simulink model "transmission"  (R2020a)
settings: Solver=ode45  StartTime=0.0  StopTime=30.0  MaxStep=0.05  RelTol=1e-3  EnableMultiTasking=on
model workspace (MAT data in the model file):
  Cd = 0.02
  F = 40
  Ie = 0.0219914882836
  Iv = 12.0941478573
  K = [137.465208994; 137.065019157; 135.864449646; 135.664354728; 137.565256453; 140.366585312; 145.268910814; 152.872517717; 162.9773111; 164.27792807; 166.178829795; 167.979684062; 170.080680706; 172.781962105; 175.383196045; 179.585189333; 183.587087703; 189.890077635; 197.693779455; 215.902417037; 244.515990379]
  Ne = [800 1200 1600 2000 2400 2800 3200 3600 4000 4400 4800]
  Qfd = 3.23
  Qn = [0; 0.1; 0.2; 0.3; 0.4; 0.5; 0.6; 0.7; 0.8; 0.81; 0.82; 0.83; 0.84; 0.85; 0.86; 0.87; 0.88; 0.89; 0.9; 0.92; 0.94]
  Qt = [2.232; 2.075; 1.975; 1.846; 1.72; 1.564; 1.409; 1.254; 1.096; 1.08; 1.061; 1.043; 1.028; 1.012; 1.002; 1.002; 1.001; 0.998; 0.999; 1.001; 1.002]
  Rw = 1
  TH = [0; 20; 30; 40; 50; 60; 70; 80; 90; 100]
  THdown = [0; 5; 40; 50; 90; 100]
  THup = [0; 25; 35; 50; 90; 100]
  Te = [-40  -44  -49  -53  -57  -61  -65  -70  -74  -78  -82; 215  117  85  66  44  29  10  -2  -13  -22  -32; 245  208  178  148  122  104  85  66  48  33  18; 264  260  241  219  193  167  152  133  119  96  85; 264  279  282  275  260  238  223  208  189  171  152; 267  290  293  297  290  275  260  256  234  212  193; 267  297  305  305  305  301  293  282  267  249  226; 267  301  308  312  319  323  319  316  297  279  253; 267  301  312  319  327  327  327  327  312  293  267; 267  301  312  319  327  334  334  334  319  305  275]
  Vdown = [0  5  20  35; 0  5  20  35; 0  5  25  40; 0  5  30  50; 0  30  50  80; 0  30  50  80]
  Vup = [10  30  50  1000000; 10  30  50  1000000; 15  30  50  1000000; 23  41  60  1000000; 40  70  100  1000000; 40  70  100  1000000]
undefined symbols (not defined in the file): sigbuilder_block
settings Model: Creator=oqaqish  LastModifiedBy=Shubham
settings DataIOCC: LimitDataPoints=on  SaveFormat=Array  ReturnWorkspaceOutputs=off  SignalLoggingName=sigsOut
settings OptimizationCC: ExpressionDepthLimit=2147483647  InitFltsAndDblsToZero=on  LifeSpan=inf
settings DebuggingCC: SaveWithParameterizedLinksMsg=none  UnderspecifiedInitializationDetection=Classic  MergeDetectMultiDrivingBlocksExec=none  CheckExecutionContextPreStartOutputMsg=on  CheckExecutionContextRuntimeOutputMsg=on  SignalResolutionControl=TryResolveAllWithWarning  MultiTaskDSMMsg=warning  MultiTaskCondExecSysMsg=none  ParameterPrecisionLossMsg=none  FcnCallInpInsideContextMsg=warning  AllowSymbolicDim=off  StateNameClashWarn=warning  SFUnexpectedBacktrackingDiag=warning  SFNoUnconditionalDefaultTransitionDiag=warning  SFExecutionAtInitializationDiag=none  ArithmeticOperatorsInVariantConditions=warning
settings HardwareCC: ProdBitPerPointer=32  ProdBitPerSizeT=32  ProdBitPerPtrDiffT=32  ProdLargestAtomicFloat=None  ProdIntDivRoundTo=Undefined  ProdEndianess=Unspecified  ProdWordSize=32  ProdHWDeviceType=32-bit Generic  TargetUnknown=on
settings ModelReferenceCC: PropagateSignalLabelsOutOfModel=off
settings SFSimCC: SimUseLocalCustomCode=off  SimParseCustomCode=off
settings RTWCC: RTWUseLocalCustomCode=off
settings CodeAppCC: StateflowObjectComments=on
settings GRTTargetCC: TargetFcnLib=ansi_tfl_tmw.mat  TargetLangStandard=C89/C90 (ANSI)  ModelReferenceCompliant=off  CombineOutputUpdateFcns=off  MatFileLogging=off  GRTInterface=on
settings ConfigComp: CovMetricSettings=dw  CovHtmlReporting=on  CovSaveCumulativeToWorkspaceVar=on  CovSaveSingleToWorkspaceVar=on  CovExternalEMLEnable=off  CovSFcnEnable=off

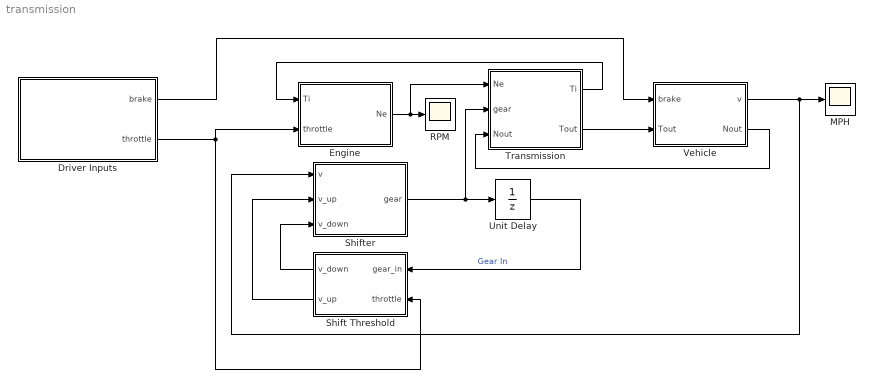
== system transmission ==
  Driver Inputs : Subsystem  Tag=STV Subsys  LoadFcn=sigbuilder_block('load');  StartFcn=sigbuilder_block('start');  StopFcn=sigbuilder_block('stop');  ClipboardFcn=sigbuilder_block('clipboard');  mask(Sigbuilder block){tuvar=[0:10]}
      mask help: Sigbuilder GUI
      mask init:
      | tuvar = sigbuilder_block('maskInit');
      settings: CopyFcn=sigbuilder_block('copy');  DeleteFcn=sigbuilder_block('delete');  ModelCloseFcn=sigbuilder_block('modelClose');  PreSaveFcn=sigbuilder_block('preSave');  PauseFcn=sigbuilder_block('pause')  ContinueFcn=sigbuilder_block('continue')  NameChangeFcn=sigbuilder_block('namechange');  OpenFcn=sigbuilder_block('open',[0 30 1152 561.6 ]);  CloseFcn=sigbuilder_block('close');
      mask Display: plot(0, 0, 100, 100,[2, 2, 32, 32, 2], [68, 8, 8, 68, 68],[32, 2], [38, 38], [32, 19, 2],[53, 60, 44], [32, 17, 17, 2],[16, 16, 31, 31]);txt = getActiveGroup(gcbh);text(2, 100, txt,'verticalAlignment', 'top');
  Engine : Subsystem
  MPH : Scope
  RPM : Scope
  Shift Threshold : Subsystem
  Shifter : Stateflow chart  TreatAsAtomicUnit=on
  Transmission : Subsystem
  Unit Delay : UnitDelay  InitialCondition=1  SampleTime=0.05  HasFrameUpgradeWarning=on
      settings: AttributesFormatString=Ts = %<SampleTime>\n
  Vehicle : Subsystem
  wires:
  Driver Inputs/2(throttle) -> Engine/2(throttle), Shift Threshold/2(throttle)
  Engine/1(Ne) -> Transmission/1(Ne), RPM/1
  Driver Inputs/1(brake) -> Vehicle/1(brake)
  Transmission/2(Tout) -> Vehicle/2(Tout)
  Unit Delay/1 -> Shift Threshold/1(gear_in)  "Gear In"
  Shift Threshold/1(v_down) -> Shifter/3(v_down)
  Shift Threshold/2(v_up) -> Shifter/2(v_up)
  Vehicle/2(Nout) -> Transmission/3(Nout)
  Vehicle/1(v) -> MPH/1, Shifter/1(v)
  Shifter/1(gear) -> Unit Delay/1, Transmission/2(gear)
  Transmission/1(Ti) -> Engine/1(Ti)

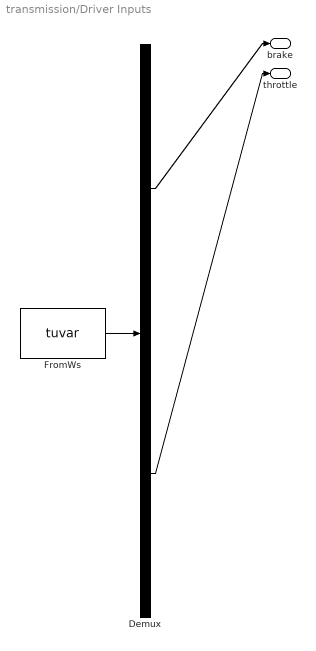
== system transmission/Driver Inputs ==
  Demux : Demux  Tag=STV Demux  Outputs=2
      settings: DisplayOption=none
  FromWs : FromWorkspace  Tag=STV FromWs  VariableName=tuvar  ZeroCross=off
      SigBuilderData=|
      | dataSet.timeRange = [0 50]
      | dataSet.name = 'Passing Maneuver'
      | sbobj.Groups.Name = 'Passing Maneuver'
      | sbobj.Groups.Signals(1).Name = 'brake'
      | sbobj.Groups.Signals(1).XData = [0 50]
      | sbobj.Groups.Signals(1).YData = [0 0]
      | sbobj.Groups.Signals(2).Name = 'throttle'
      | sbobj.Groups.Signals(2).XData = [0 15 15 50]
      | sbobj.Groups.Signals(2).YData = [60 40 100 60]
      | sbobj.Groups.TimeRange = [0 50]
  brake : Outport  Tag=STV Outport  VectorParamsAs1DForOutWhenUnconnected=off
  throttle : Outport  Tag=STV Outport  Port=2  VectorParamsAs1DForOutWhenUnconnected=off
  wires:
  Demux/2 -> throttle/1
  Demux/1 -> brake/1
  FromWs/1 -> Demux/1

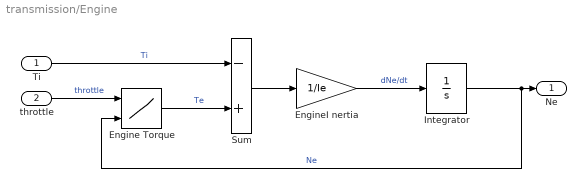
== system transmission/Engine ==
  Ti : Inport
  throttle : Inport  Port=2
  Engine Torque : Lookup2D  RowIndex=TH  ColumnIndex=Ne  Table=Te  SaturateOnIntegerOverflow=on
  EngineI nertia : Gain  Gain=1/Ie  SaturateOnIntegerOverflow=on  OutDataTypeStr=Inherit: Same as input  ParamDataTypeStr=Inherit: Same as input
  Integrator : Integrator  InitialCondition=1000  LimitOutput=on  UpperSaturationLimit=6000  LowerSaturationLimit=600  ZeroCross=off
      settings: AttributesFormatString="Ne0 = %<InitialCondition>\\n%<LowerSaturationLimit> <= Ne <=  %<UpperSaturationLimit>\\n\\n"
  Sum : Sum  Inputs=-+  InputSameDT=on  SaturateOnIntegerOverflow=on  OutDataTypeStr=Inherit: Same as first input
  Ne : Outport  VectorParamsAs1DForOutWhenUnconnected=off
  wires:
  Sum/1 -> EngineI nertia/1
  throttle/1 -> Engine Torque/1  "throttle"
  Engine Torque/1 -> Sum/2  "Te"
  Ti/1 -> Sum/1  "Ti"
  Integrator/1 -> Ne/1, Engine Torque/2  "Ne"
  EngineI nertia/1 -> Integrator/1  "dNe/dt"

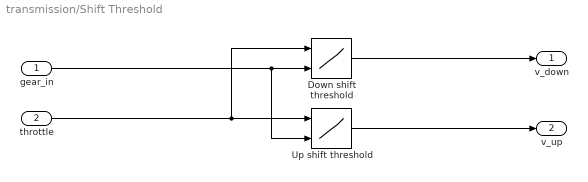
== system transmission/Shift Threshold ==
  gear_in : Inport
  throttle : Inport  Port=2
  Down shift threshold : Lookup2D  RowIndex=THdown  ColumnIndex=[1:4]  Table=Vdown  InputSameDT=on
  Up shift threshold : Lookup2D  RowIndex=THup  ColumnIndex=[1:4]  Table=Vup  InputSameDT=on
  v_down : Outport  VectorParamsAs1DForOutWhenUnconnected=off
  v_up : Outport  Port=2  VectorParamsAs1DForOutWhenUnconnected=off
  wires:
  Up shift threshold/1 -> v_up/1
  Down shift threshold/1 -> v_down/1
  throttle/1 -> Up shift threshold/1, Down shift threshold/1
  gear_in/1 -> Up shift threshold/2, Down shift threshold/2

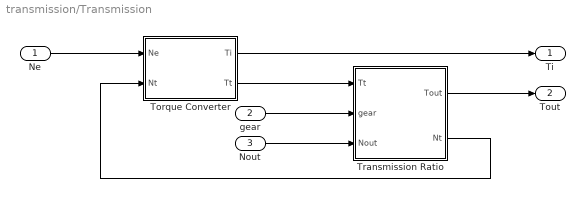
== system transmission/Transmission ==
  Ne : Inport
  gear : Inport  Port=2
  Nout : Inport  Port=3
  Torque Converter : Subsystem
  Transmission Ratio : Subsystem
  Ti : Outport  InitialOutput=0  VectorParamsAs1DForOutWhenUnconnected=off
  Tout : Outport  Port=2  InitialOutput=0  VectorParamsAs1DForOutWhenUnconnected=off
  wires:
  Transmission Ratio/2(Nt) -> Torque Converter/2(Nt)
  Ne/1 -> Torque Converter/1(Ne)
  gear/1 -> Transmission Ratio/2(gear)
  Nout/1 -> Transmission Ratio/3(Nout)
  Transmission Ratio/1(Tout) -> Tout/1
  Torque Converter/2(Tt) -> Transmission Ratio/1(Tt)
  Torque Converter/1(Ti) -> Ti/1

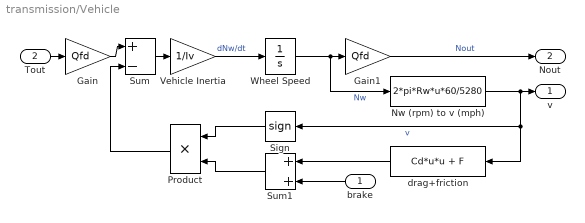
== system transmission/Vehicle ==
  brake : Inport
  Tout : Inport  Port=2
  Gain : Gain  Gain=Qfd  SaturateOnIntegerOverflow=on  OutDataTypeStr=Inherit: Same as input  ParamDataTypeStr=Inherit: Same as input
  Gain1 : Gain  Gain=Qfd  SaturateOnIntegerOverflow=on  OutDataTypeStr=Inherit: Same as input  ParamDataTypeStr=Inherit: Same as input
  Nw (rpm) to v (mph) : Fcn  Expr=2*pi*Rw*u*60/5280
  Product : Product  SaturateOnIntegerOverflow=on  OutDataTypeStr=Inherit: Same as first input
  Sign : Signum
  Sum : Sum  Inputs=|+-  SaturateOnIntegerOverflow=on
  Sum1 : Sum  SaturateOnIntegerOverflow=on
  Vehicle Inertia : Gain  Gain=1/Iv  SaturateOnIntegerOverflow=on  OutDataTypeStr=Inherit: Same as input  ParamDataTypeStr=Inherit: Same as input
  Wheel Speed : Integrator
      settings: AttributesFormatString=Nw0 = %<InitialCondition>\n
  drag+friction : Fcn  Expr=Cd*u*u + F
  v : Outport  VectorParamsAs1DForOutWhenUnconnected=off
  Nout : Outport  Port=2  VectorParamsAs1DForOutWhenUnconnected=off
  wires:
  Tout/1 -> Gain/1
  Gain/1 -> Sum/1
  Sum/1 -> Vehicle Inertia/1
  Wheel Speed/1 -> Gain1/1, Nw (rpm) to v (mph)/1  "Nw"
  Gain1/1 -> Nout/1  "Nout"
  Nw (rpm) to v (mph)/1 -> v/1, Sign/1, drag+friction/1  "v"
  Vehicle Inertia/1 -> Wheel Speed/1  "dNw/dt"
  brake/1 -> Sum1/2
  drag+friction/1 -> Sum1/1
  Sign/1 -> Product/1
  Sum1/1 -> Product/2
  Product/1 -> Sum/2

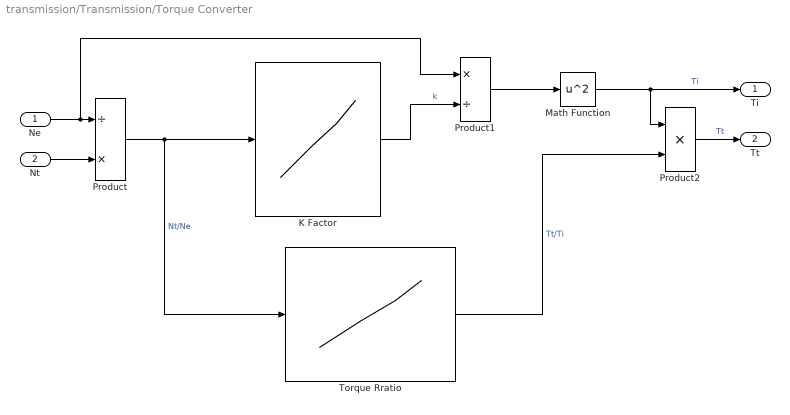
== system transmission/Transmission/Torque Converter ==
  Ne : Inport
  Nt : Inport  Port=2
  K Factor : Lookup  InputValues=Qn  Table=K  SaturateOnIntegerOverflow=on
  Math Function : Math  Operator=square  SignedPower=on  SaturateOnIntegerOverflow=on
  Product : Product  Inputs=/*  SaturateOnIntegerOverflow=on  OutDataTypeStr=Inherit: Same as first input
  Product1 : Product  Inputs=*/  SaturateOnIntegerOverflow=on  OutDataTypeStr=Inherit: Same as first input
  Product2 : Product  Inputs=**  SaturateOnIntegerOverflow=on  OutDataTypeStr=Inherit: Same as first input
  Torque Rratio : Lookup  InputValues=Qn  Table=Qt  SaturateOnIntegerOverflow=on
  Ti : Outport  VectorParamsAs1DForOutWhenUnconnected=off
  Tt : Outport  Port=2  VectorParamsAs1DForOutWhenUnconnected=off
  wires:
  Product1/1 -> Math Function/1
  Torque Rratio/1 -> Product2/2  "Tt/Ti"
  Math Function/1 -> Product2/1, Ti/1  "Ti"
  K Factor/1 -> Product1/2  "k"
  Product/1 -> K Factor/1, Torque Rratio/1  "Nt/Ne"
  Ne/1 -> Product1/1, Product/1
  Product2/1 -> Tt/1  "Tt"
  Nt/1 -> Product/2

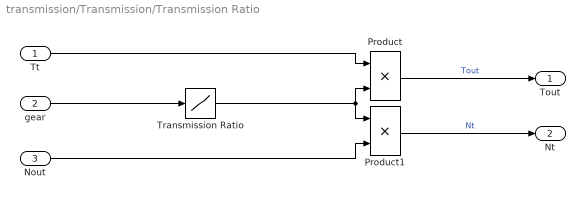
== system transmission/Transmission/Transmission Ratio ==
  Tt : Inport
  gear : Inport  Port=2
  Nout : Inport  Port=3
  Product : Product  InputSameDT=on  SaturateOnIntegerOverflow=on  OutDataTypeStr=Inherit: Same as first input
  Product1 : Product  InputSameDT=on  SaturateOnIntegerOverflow=on  OutDataTypeStr=Inherit: Same as first input
  Transmission Ratio : Lookup  InputValues=[1, 2, 3, 4]  Table=[2.393, 1.450, 1.000, 0.677]  SaturateOnIntegerOverflow=on
  Tout : Outport  InitialOutput=0  VectorParamsAs1DForOutWhenUnconnected=off
  Nt : Outport  Port=2  InitialOutput=0  VectorParamsAs1DForOutWhenUnconnected=off
  wires:
  gear/1 -> Transmission Ratio/1
  Tt/1 -> Product/1
  Product/1 -> Tout/1  "Tout"
  Product1/1 -> Nt/1  "Nt"
  Nout/1 -> Product1/2
  Transmission Ratio/1 -> Product1/1, Product/2

== stateflow chart transmission/Shifter ==
  settings: updateMethod=DISCRETE  sampleTime=0.05
  state gear4
    en: gear = 4;
  state gear1
    en: gear = 1;
  state gear2
    en: gear = 2;
  state gear3
    en: gear = 3;
  (default) -> gear1
  gear2 -> gear3 [order 1] : [v > v_up]
  gear3 -> gear4 [order 1] : [v > v_up]
  gear1 -> gear2 : [v > v_up]
  gear4 -> gear3 : [v < v_down]
  gear3 -> gear2 [order 2] : [v < v_down]
  gear2 -> gear1 [order 2] : [v < v_down]
  data: v input double; v_up input double; v_down input double; gear output double
